simulink model "practico_1_modelo"  (R2021b)
settings: Solver=VariableStepAuto  StartTime=0.0  StopTime=60  RelTol=1e-3
values from neighbouring files (symbols this model uses):
  A_d = exp(dfdh_eval*Ts)    [p1_code.m]
  B_d = dfdh_eval^(-1) * (A_d-1) * dfdk_eval    [p1_code.m]
  F_in = 0.0035    [p1_code.m]
  F_out = a*sqrt(2*g)    [p1_code.m]
  h_bar = 0.2    [p1_code.m]
  k_bar = F_in / (a*sqrt(2*9.81*h_bar))    [p1_code.m]
  k_list = [0.05, 0.15, 0.30, 0.50, 0.90]    [p1_code.m]
  r_0 = 0.05    [p1_code.m]
  theta = 60    [p1_code.m]
  Ts = 1    [p1_code.m]
undefined symbols (not defined in the file or in its folder): den, num
settings Model: Creator=trulscarlson  LastModifiedBy=trulscarlson

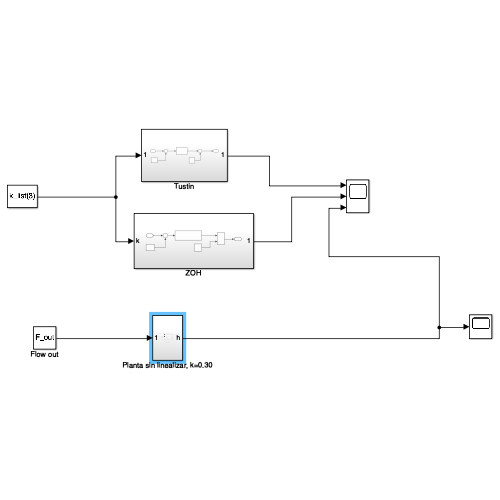
[thumbnail: Simulink's stored preview of the top-level diagram]
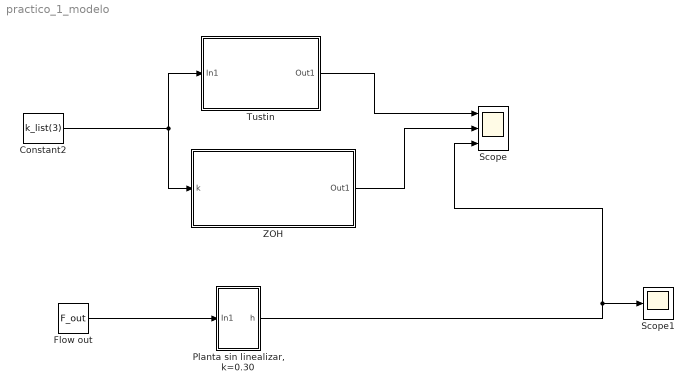
== system practico_1_modelo ==
  Constant2 : Constant  Value=k_list(3)
  Flow out : Constant  Value=F_out
  "Planta sin linealizar, k=0.30" : Subsystem
  Scope : Scope  NumInputPorts=3
  Scope1 : Scope
  Tustin : Subsystem
  ZOH : Subsystem
  wires:
  Flow out/1 -> "Planta sin linealizar, k=0.30"/1(In1)
  "Planta sin linealizar, k=0.30"/1(h) -> Scope1/1, Scope/3
  Constant2/1 -> ZOH/1(k), Tustin/1(In1)
  Tustin/1(Out1) -> Scope/1
  ZOH/1(Out1) -> Scope/2

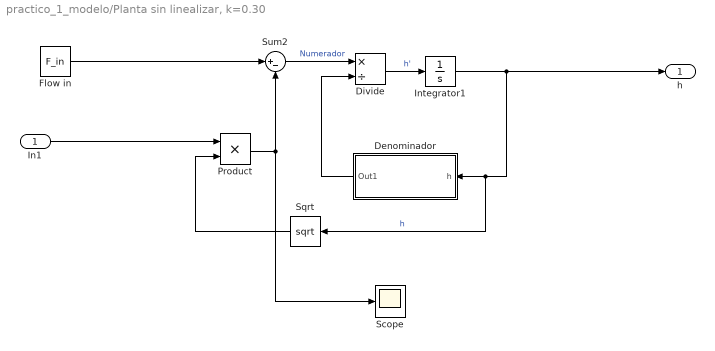
== system practico_1_modelo/Planta sin linealizar, k=0.30 ==
  In1 : Inport
  Denominador : Subsystem
  Divide : Product  Inputs=*/
  Flow in : Constant  Value=F_in
  Integrator1 : Integrator  InitialCondition=h_bar
  Product : Product
  Scope : Scope
  Sqrt : Sqrt  SaturateOnIntegerOverflow=on
  Sum2 : Sum  Inputs=|+-
  h : Outport
  wires:
  Product/1 -> Scope/1, Sum2/2
  Flow in/1 -> Sum2/1
  Divide/1 -> Integrator1/1  "h'"
  In1/1 -> Product/1
  Denominador/1(Out1) -> Divide/2
  Integrator1/1 -> h/1, Sqrt/1, Denominador/1(h)  "h"
  Sum2/1 -> Divide/1  "Numerador"
  Sqrt/1 -> Product/2

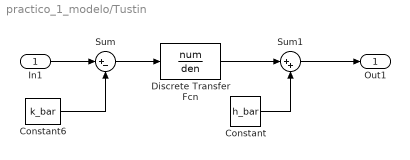
== system practico_1_modelo/Tustin ==
  In1 : Inport
  Constant : Constant  Value=h_bar
  Constant6 : Constant  Value=k_bar
  Discrete Transfer Fcn : DiscreteTransferFcn  Numerator=num  Denominator=den  SampleTime=2
  Sum : Sum  Inputs=|+-
  Sum1 : Sum  Inputs=|++
  Out1 : Outport
  wires:
  Sum1/1 -> Out1/1
  Constant/1 -> Sum1/2
  Constant6/1 -> Sum/2
  Sum/1 -> Discrete Transfer Fcn/1
  Discrete Transfer Fcn/1 -> Sum1/1
  In1/1 -> Sum/1

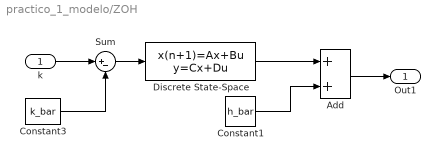
== system practico_1_modelo/ZOH ==
  k : Inport
  Add : Sum
  Constant1 : Constant  Value=h_bar
  Constant3 : Constant  Value=k_bar
  Discrete State-Space : DiscreteStateSpace  A=A_d  B=B_d  D=0  SampleTime=Ts
  Sum : Sum  Inputs=|+-
  Out1 : Outport
  wires:
  k/1 -> Sum/1
  Constant3/1 -> Sum/2
  Sum/1 -> Discrete State-Space/1
  Constant1/1 -> Add/2
  Discrete State-Space/1 -> Add/1
  Add/1 -> Out1/1

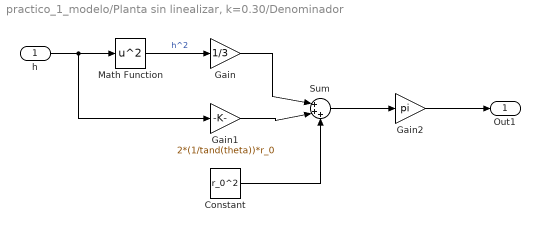
== system practico_1_modelo/Planta sin linealizar, k=0.30/Denominador ==
  h : Inport
  Constant : Constant  Value=r_0^2
  Gain : Gain  Gain=1/3
  Gain1 : Gain  Gain=2*(1/tand(theta))*r_0
  Gain2 : Gain  Gain=pi
  Math Function : Math  Operator=square  SaturateOnIntegerOverflow=on
  Sum : Sum  Inputs=|+++
  Out1 : Outport
  wires:
  h/1 -> Gain1/1, Math Function/1
  Math Function/1 -> Gain/1  "h^2"
  Gain/1 -> Sum/1
  Gain1/1 -> Sum/2
  Constant/1 -> Sum/3
  Sum/1 -> Gain2/1
  Gain2/1 -> Out1/1
